simulink model "sampleModel1716"  (R2023a)
settings: Solver=VariableStepAuto  StartTime=0.0  StopTime=10.0  RelTol=1e-3
libraries: hdlsllib x4, simulink x3
settings Model: Creator=user1  LastModifiedBy=user1

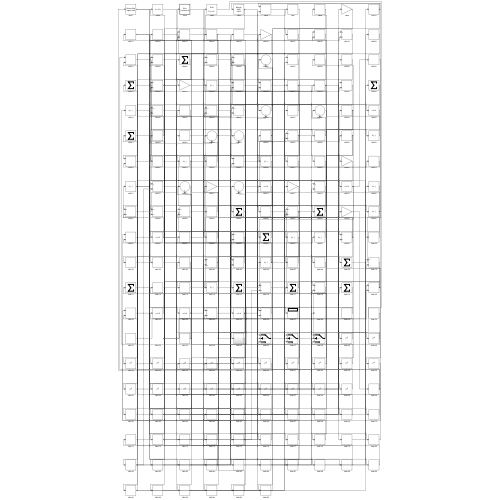
[thumbnail: Simulink's stored preview of the top-level diagram]
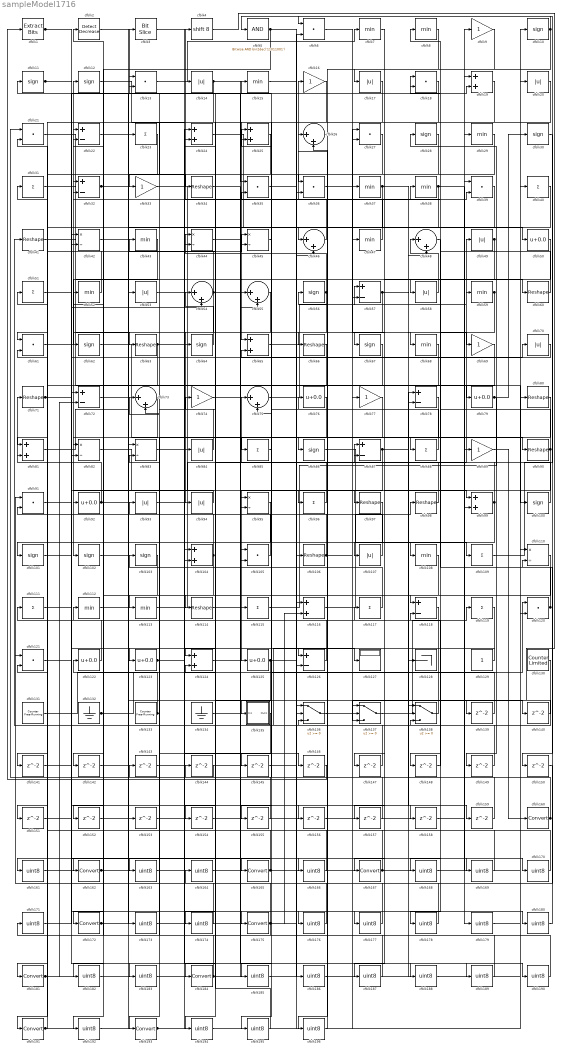
== system sampleModel1716 ==
  cfblk1 : simulink/Logic and Bit Operations/Extract Bits  bitsToExtract=Upper half  numBits=8  bitIdxRange=[0 7]  outScalingMode=Preserve fixed-point scaling
      settings: LibrarySourceBlock=|
      | hdlsllib/Logic and Bit
      | Operations/Extract Bits
  cfblk{10..12,28,30,56,62,64,67,86,100..103} (14 alike) : Signum
  cfblk{19,24..25,65,81,99,104,116,124} (9 alike) : Sum
  cfblk{6,13,18,21,27,35..36,39,61,91,105,120..121} (13 alike) : DotProduct  OutDataTypeStr=Inherit: Inherit via internal rule
  cfblk{34,41,60,63,66,71,80,90,97..98,106,114} (12 alike) : Reshape
  cfblk{14,17,20,49,53,58,70,84,93..94,107} (11 alike) : Abs  SaturateOnIntegerOverflow=off
  cfblk{7..8,15,29,37..38,43,47,52,59,68,108,112..113} (14 alike) : MinMax
  cfblk{23,31,40,51,85,88,96,109,111,115,117,119} (12 alike) : Sum  Inputs=+
  cfblk{42,44..45,82..83,95,110} (7 alike) : Product  Inputs=*/  RndMeth=Zero  SaturateOnIntegerOverflow=on
  cfblk{22,32,57,72,78,87,118,126} (8 alike) : Sum  Inputs=+-
  cfblk{50,76,79,92,122..123,125} (7 alike) : Bias  Bias=0.0  SaturateOnIntegerOverflow=off
  cfblk127 : Display
  cfblk128 : Terminator
  cfblk129 : Constant  SampleTime=-1
  cfblk130 : hdlsllib/Sources/Counter Limited  uplimit=7  tsamp=-1
  cfblk131 : hdlsllib/Sources/Counter Free-Running  NumBits=16  tsamp=-1
  cfblk132 : Ground
  cfblk133 : hdlsllib/Sources/Counter Free-Running  NumBits=16  tsamp=-1
  cfblk134 : Ground
  cfblk135 : Subsystem
      settings: LibrarySourceBlock=|
      | hdlsllib/Ports &
      | Subsystems/Subsystem
  cfblk136 : Switch  SaturateOnIntegerOverflow=off  InputSameDT=off
  cfblk137 : Switch  SaturateOnIntegerOverflow=off  InputSameDT=off
  cfblk138 : Switch  SaturateOnIntegerOverflow=off  InputSameDT=off
  cfblk{139..159} (21 alike) : Delay  SampleTime=1
  cfblk{9,16,33,69,74,77,89} (7 alike) : Gain
  cfblk{160,162,165,167,172,175,181,184,191,193} (10 alike) : DataTypeConversion  SaturateOnIntegerOverflow=off  RndMeth=Floor
  cfblk{161,163..164,166,168..171,173..174,176..180,182..183,185..190,192,194..196} (27 alike) : DataTypeConversion  OutDataTypeStr=uint8  SaturateOnIntegerOverflow=off  RndMeth=Floor
  cfblk2 : simulink/Logic and Bit Operations/Detect Decrease  vinit=0.0  OutDataTypeStr=boolean
      settings: LibrarySourceBlock=|
      | hdlsllib/Logic and Bit
      | Operations/Detect
      | Decrease
  cfblk{26,46,48,54..55,73,75} (7 alike) : Sum  Inputs=|++
  cfblk3 : hdlsllib/Logic and Bit Operations/Bit Slice  lidx=7  ridx=0
  cfblk4 : ArithShift  BitShiftNumber=8
  cfblk5 : simulink/Logic and Bit Operations/Bitwise Operator  logicop=AND  UseBitMask=on  BitMask=bin2dec('11011001')  BitMaskRealWorld=Stored Integer
      settings: LibrarySourceBlock=|
      | hdlsllib/Logic and Bit
      | Operations/Bitwise
      | Operator
  wires:
  cfblk20/1 -> cfblk65/1
  cfblk47/1 -> cfblk16/1
  cfblk51/1 -> cfblk165/1
  cfblk113/1 -> cfblk49/1
  cfblk55/1 -> cfblk94/1
  cfblk115/1 -> cfblk28/1
  cfblk33/1 -> cfblk125/1
  cfblk56/1 -> cfblk44/1, cfblk62/1
  cfblk67/1 -> cfblk135/1(In1)
  cfblk61/1 -> cfblk3/1
  cfblk116/1 -> cfblk98/1
  cfblk75/1 -> cfblk59/1
  cfblk86/1 -> cfblk109/1
  cfblk13/1 -> cfblk7/1
  cfblk65/1 -> cfblk57/1
  cfblk104/1 -> cfblk2/1, cfblk142/1
  cfblk27/1 -> cfblk162/1
  cfblk119/1 -> cfblk41/1
  cfblk96/1 -> cfblk75/1
  cfblk92/1 -> cfblk71/1, cfblk45/1, cfblk15/1
  cfblk43/1 -> cfblk102/1
  cfblk62/1 -> cfblk90/1
  cfblk45/1 -> cfblk85/1
  cfblk118/1 -> cfblk117/1
  cfblk109/1 -> cfblk6/1
  cfblk131/1 -> cfblk120/1
  cfblk15/1 -> cfblk60/1
  cfblk87/1 -> cfblk115/1, cfblk159/1
  cfblk46/1 -> cfblk4/1
  cfblk6/1 -> cfblk68/1
  cfblk99/1 -> cfblk26/2, cfblk114/1, cfblk87/2
  cfblk54/1 -> cfblk126/2, cfblk31/1, cfblk152/1
  cfblk77/1 -> cfblk193/1
  cfblk18/1 -> cfblk33/1
  cfblk11/1 -> cfblk123/1, cfblk127/1
  cfblk129/1 -> cfblk126/1
  cfblk50/1 -> cfblk107/1
  cfblk90/1 -> cfblk18/2, cfblk157/1
  cfblk70/1 -> cfblk65/2
  cfblk137/1 -> cfblk119/1
  cfblk84/1 -> cfblk13/1
  cfblk2/1 -> cfblk97/1
  cfblk49/1 -> cfblk108/1, cfblk148/1
  cfblk69/1 -> cfblk101/1
  cfblk132/1 -> cfblk20/1, cfblk116/1
  cfblk31/1 -> cfblk100/1
  cfblk57/1 -> cfblk69/1, cfblk194/1
  cfblk107/1 -> cfblk93/1
  cfblk122/1 -> cfblk21/2
  cfblk120/1 -> cfblk8/1, cfblk113/1
  cfblk134/1 -> cfblk18/1
  cfblk36/1 -> cfblk37/1
  cfblk73/1 -> cfblk172/1
  cfblk1/1 -> cfblk99/1, cfblk54/2
  cfblk136/1 -> cfblk57/2
  cfblk93/1 -> cfblk38/1
  cfblk71/1 -> cfblk70/1, cfblk166/1
  cfblk12/1 -> cfblk84/1
  cfblk16/1 -> cfblk124/1
  cfblk94/1 -> cfblk92/1
  cfblk39/1 -> cfblk64/1
  cfblk121/1 -> cfblk175/1
  cfblk64/1 -> cfblk54/1
  cfblk24/1 -> cfblk46/1
  cfblk81/1 -> cfblk53/1
  cfblk22/1 -> cfblk34/1
  cfblk117/1 -> cfblk103/1
  cfblk126/1 -> cfblk112/1
  cfblk21/1 -> cfblk63/1
  cfblk53/1 -> cfblk58/1
  cfblk133/1 -> cfblk43/1, cfblk22/2
  cfblk52/1 -> cfblk22/1
  cfblk78/1 -> cfblk184/1
  cfblk123/1 -> cfblk104/2, cfblk83/2
  cfblk9/1 -> cfblk86/1
  cfblk7/1 -> cfblk67/1
  cfblk88/1 -> cfblk11/1
  cfblk82/1 -> cfblk136/1
  cfblk28/1 -> cfblk66/1
  cfblk68/1 -> cfblk96/1
  cfblk125/1 -> cfblk25/1, cfblk87/1, cfblk174/1
  cfblk37/1 -> cfblk138/1, cfblk45/2
  cfblk14/1 -> cfblk35/1, cfblk81/1, cfblk61/1
  cfblk63/1 -> cfblk82/2, cfblk140/1
  cfblk8/1 -> cfblk17/1
  cfblk79/1 -> cfblk30/1, cfblk149/1
  cfblk38/1 -> cfblk151/1, cfblk170/1
  cfblk95/1 -> cfblk181/1
  cfblk23/1 -> cfblk191/1
  cfblk58/1 -> cfblk48/1
  cfblk60/1 -> cfblk32/1
  cfblk100/1 -> cfblk25/2
  cfblk5/1 -> cfblk82/1, cfblk48/2
  cfblk138/1 -> cfblk32/2
  cfblk29/1 -> cfblk167/1
  cfblk91/1 -> cfblk19/2
  cfblk72/1 -> cfblk137/3
  cfblk32/1 -> cfblk79/1, cfblk50/1
  cfblk17/1 -> cfblk105/1
  cfblk105/1 -> cfblk14/1
  cfblk106/1 -> cfblk39/2, cfblk52/1, cfblk81/2
  cfblk89/1 -> cfblk160/1
  cfblk41/1 -> cfblk55/1
  cfblk10/1 -> cfblk36/1, cfblk5/1
  cfblk59/1 -> cfblk118/1, cfblk88/1
  cfblk98/1 -> cfblk24/2
  cfblk130/1 -> cfblk138/3
  cfblk4/1 -> cfblk139/1
  cfblk139/1 -> cfblk75/2
  cfblk140/1 -> cfblk137/2
  cfblk97/1 -> cfblk141/1
  cfblk141/1 -> cfblk72/1
  cfblk142/1 -> cfblk6/2
  cfblk143/1 -> cfblk105/2
  cfblk144/1 -> cfblk21/1
  cfblk80/1 -> cfblk145/1
  cfblk145/1 -> cfblk136/2
  cfblk3/1 -> cfblk146/1
  cfblk146/1 -> cfblk1/1
  cfblk108/1 -> cfblk147/1
  cfblk147/1 -> cfblk13/2
  cfblk148/1 -> cfblk118/2
  cfblk149/1 -> cfblk44/2
  cfblk30/1 -> cfblk150/1
  cfblk152/1 -> cfblk19/1
  cfblk112/1 -> cfblk153/1
  cfblk153/1 -> cfblk138/2
  cfblk25/1 -> cfblk154/1
  cfblk154/1 -> cfblk99/2
  cfblk85/1 -> cfblk155/1
  cfblk155/1 -> cfblk91/2
  cfblk101/1 -> cfblk156/1
  cfblk156/1 -> cfblk26/1
  cfblk157/1 -> cfblk137/1
  cfblk34/1 -> cfblk158/1
  cfblk159/1 -> cfblk124/2
  cfblk160/1 -> cfblk136/3, cfblk35/2
  cfblk161/1 -> cfblk89/1
  cfblk162/1 -> cfblk128/1, cfblk9/1
  cfblk135/1(Out1) -> cfblk163/1
  cfblk163/1 -> cfblk27/1
  cfblk150/1 -> cfblk164/1
  cfblk164/1 -> cfblk27/2
  cfblk165/1 -> cfblk161/1, cfblk12/1
  cfblk166/1 -> cfblk51/1
  cfblk167/1 -> cfblk80/1, cfblk83/1
  cfblk48/1 -> cfblk168/1
  cfblk168/1 -> cfblk29/1
  cfblk42/1 -> cfblk169/1
  cfblk169/1 -> cfblk39/1
  cfblk170/1 -> cfblk42/1
  cfblk171/1 -> cfblk42/2
  cfblk172/1 -> cfblk46/2, cfblk106/1
  cfblk102/1 -> cfblk173/1
  cfblk173/1 -> cfblk73/1
  cfblk174/1 -> cfblk73/2
  cfblk175/1 -> cfblk171/1, cfblk116/2, cfblk91/1
  cfblk74/1 -> cfblk176/1
  cfblk176/1 -> cfblk121/1
  cfblk114/1 -> cfblk177/1
  cfblk177/1 -> cfblk121/2
  cfblk110/1 -> cfblk178/1
  cfblk178/1 -> cfblk56/1
  cfblk158/1 -> cfblk179/1
  cfblk179/1 -> cfblk110/1
  cfblk124/1 -> cfblk180/1
  cfblk180/1 -> cfblk110/2
  cfblk181/1 -> cfblk55/2, cfblk10/1, cfblk72/2
  cfblk19/1 -> cfblk182/1
  cfblk182/1 -> cfblk95/1
  cfblk151/1 -> cfblk183/1
  cfblk183/1 -> cfblk95/2
  cfblk184/1 -> cfblk143/1, cfblk104/1
  cfblk66/1 -> cfblk185/1
  cfblk185/1 -> cfblk78/1
  cfblk35/1 -> cfblk186/1
  cfblk186/1 -> cfblk78/2
  cfblk40/1 -> cfblk187/1
  cfblk187/1 -> cfblk144/1
  cfblk83/1 -> cfblk188/1
  cfblk188/1 -> cfblk40/1
  cfblk111/1 -> cfblk189/1
  cfblk189/1 -> cfblk122/1
  cfblk44/1 -> cfblk190/1
  cfblk190/1 -> cfblk111/1
  cfblk191/1 -> cfblk61/2, cfblk47/1, cfblk24/1
  cfblk103/1 -> cfblk192/1
  cfblk192/1 -> cfblk23/1
  cfblk193/1 -> cfblk36/2, cfblk120/2
  cfblk194/1 -> cfblk77/1
  cfblk76/1 -> cfblk195/1
  cfblk195/1 -> cfblk74/1
  cfblk26/1 -> cfblk196/1
  cfblk196/1 -> cfblk76/1

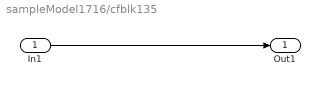
== system sampleModel1716/cfblk135 ==
  In1 : Inport
  Out1 : Outport
  wires:
  In1/1 -> Out1/1
